simulink model "corr_hw_test"  (R2012b)
settings: Solver=ode45  StartTime=0.0  StopTime=200000  RelTol=1e-3
undefined symbols (not defined in the file or in its folder): gcbh, sfp, xlBlockLoadCallback
libraries: xbsIndex_r4 x1902, casper_library_misc x15, xps_library x6, ox_lib x1
(part 6 of 16)

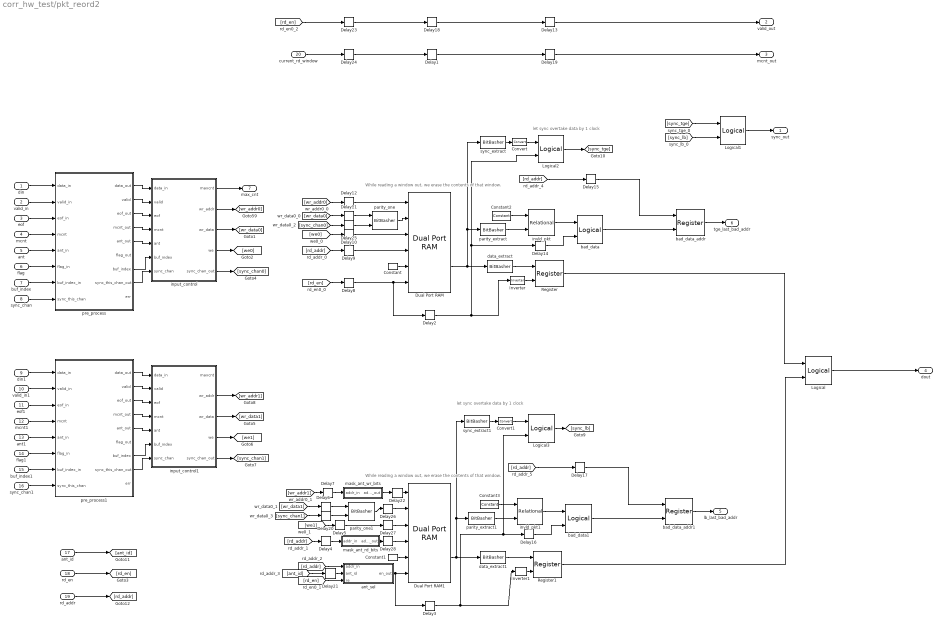
== system corr_hw_test/pkt_reord2 ==
  note: let sync overtake data by 1 clock
  note: While reading a window out,
      | we erase the contents of that window.
  note: While reading a window out,
      | we erase the contents of that window.
  note: let sync overtake data by 1 clock
  din : Inport
  valid_in : Inport  Port=2
  eof : Inport  Port=3
  mcnt : Inport  Port=4
  ant : Inport  Port=5
  flag : Inport  Port=6
  buf_index : Inport  Port=7
  sync_chan : Inport  Port=8
  din1 : Inport  Port=9
  valid_in1 : Inport  Port=10
  eof1 : Inport  Port=11
  mcnt1 : Inport  Port=12
  ant1 : Inport  Port=13
  flag1 : Inport  Port=14
  buf_index1 : Inport  Port=15
  sync_chan1 : Inport  Port=16
  ant_id : Inport  Port=17
  rd_en : Inport  Port=18
  rd_addr : Inport  Port=19
  current_rd_window : Inport  Port=20
  Constant : xbsIndex_r4/Constant  const=0  gui_display_data_type=Fixed-point  arith_type=Unsigned  n_bits=9*(2^x_parallel_bits)  bin_pt=0  preci_type=Single  exp_width=8  frac_width=24  explicit_period=on  period=1  equ=P=C  opselect=C  inp2=PCIN>>17  opr=+  inp1=P  carry=CIN  dbl_ovrd=off  block_type=constant
  Constant1 : xbsIndex_r4/Constant  const=0  gui_display_data_type=Fixed-point  arith_type=Unsigned  n_bits=9*(2^x_parallel_bits)  bin_pt=0  preci_type=Single  exp_width=8  frac_width=24  explicit_period=on  period=1  equ=P=C  opselect=C  inp2=PCIN>>17  opr=+  inp1=P  carry=CIN  dbl_ovrd=off  block_type=constant
  Constant2 : xbsIndex_r4/Constant  const=3  gui_display_data_type=Fixed-point  arith_type=Unsigned  n_bits=2  bin_pt=0  preci_type=Single  exp_width=8  frac_width=24  explicit_period=on  period=1  equ=P=C  opselect=C  inp2=PCIN>>17  opr=+  inp1=P  carry=CIN  dbl_ovrd=off  block_type=constant
  Constant3 : xbsIndex_r4/Constant  const=1  gui_display_data_type=Fixed-point  arith_type=Unsigned  n_bits=1  bin_pt=0  preci_type=Single  exp_width=8  frac_width=24  explicit_period=on  period=1  equ=P=C  opselect=C  inp2=PCIN>>17  opr=+  inp1=P  carry=CIN  dbl_ovrd=off  block_type=constant
  Convert : xbsIndex_r4/Convert  gui_display_data_type=Boolean  arith_type=Boolean  n_bits=3  bin_pt=0  float_type=Single  exp_bits=8  fraction_bits=24  quantization=Truncate  overflow=Wrap  en=off  latency=0  dbl_ovrd=off  pipeline=off  block_type=convert
      settings: block_version=11.4
  Convert1 : xbsIndex_r4/Convert  gui_display_data_type=Boolean  arith_type=Boolean  n_bits=3  bin_pt=0  float_type=Single  exp_bits=8  fraction_bits=24  quantization=Truncate  overflow=Wrap  en=off  latency=0  dbl_ovrd=off  pipeline=off  block_type=convert
      settings: block_version=11.4
  Delay{1..3,18} (4 alike) : xbsIndex_r4/Delay  rst=off  infoeditControl=Selection of Reset will increase slice count due to use of real FFs and instead of SRLs  en=off  latency=3  dbl_ovrd=off  reg_retiming=on  block_type=delay
      settings: xl_area=[0, 0, 0, 0, 0, 0, 0]
  Delay{4..13,19..20,23..25} (15 alike) : xbsIndex_r4/Delay  rst=off  infoeditControl=Selection of Reset will increase slice count due to use of real FFs and instead of SRLs  en=off  latency=1  dbl_ovrd=off  reg_retiming=on  block_type=delay
      settings: xl_area=[0, 0, 0, 0, 0, 0, 0]
  Delay{14,16,21..22,26..28} (7 alike) : xbsIndex_r4/Delay  rst=off  infoeditControl=Selection of Reset will increase slice count due to use of real FFs and instead of SRLs  en=off  latency=1  dbl_ovrd=off  reg_retiming=off  block_type=delay
      settings: xl_area=[0, 0, 0, 0, 0, 0, 0]
  Delay15 : xbsIndex_r4/Delay  rst=off  infoeditControl=Selection of Reset will increase slice count due to use of real FFs and instead of SRLs  en=off  latency=5  dbl_ovrd=off  reg_retiming=on  block_type=delay
      settings: xl_area=[0, 0, 0, 0, 0, 0, 0]
  Delay17 : xbsIndex_r4/Delay  rst=off  infoeditControl=Selection of Reset will increase slice count due to use of real FFs and instead of SRLs  en=off  latency=5  dbl_ovrd=off  reg_retiming=on  block_type=delay
      settings: xl_area=[0, 0, 0, 0, 0, 0, 0]
  Dual Port RAM : xbsIndex_r4/Dual Port RAM  depth=2^x_int_bits * 2^ant_bits * 2^window_bits * 2^(x_parallel_bits - 3)  initVector=1  distributed_mem=Block RAM  init_a=0  init_b=0  rst_a=off  rst_b=off  en_a=off  en_b=off  latency=3  write_mode_A=Read Before Write  write_mode_B=Read Before Write  dbl_ovrd=off  optimize=Area  block_type=dpram
      settings: xl_area=[0, 0, 0, 0, 0, 0, 0]  block_version=10.1.3
  Dual Port RAM1 : xbsIndex_r4/Dual Port RAM  depth=2^x_int_bits * 2^window_bits * 2^(x_parallel_bits - 3)  initVector=1  distributed_mem=Block RAM  init_a=0  init_b=0  rst_a=off  rst_b=off  en_a=off  en_b=off  latency=3  write_mode_A=Read Before Write  write_mode_B=Read Before Write  dbl_ovrd=off  optimize=Area  block_type=dpram
      settings: xl_area=[0, 0, 0, 0, 0, 0, 0]  block_version=10.1.3
  Inverter : xbsIndex_r4/Inverter  en=off  latency=0  dbl_ovrd=off  block_type=inv
  Inverter1 : xbsIndex_r4/Inverter  en=off  latency=0  dbl_ovrd=off  block_type=inv
  Logical : xbsIndex_r4/Logical  logical_function=OR  inputs=2  en=off  latency=0  precision=Full  arith_type=Unsigned  n_bits=16  bin_pt=0  align_bp=on  dbl_ovrd=off  block_type=logical
  Logical1 : xbsIndex_r4/Logical  logical_function=OR  inputs=2  en=off  latency=0  precision=Full  arith_type=Unsigned  n_bits=16  bin_pt=0  align_bp=on  dbl_ovrd=off  block_type=logical
  Logical2 : xbsIndex_r4/Logical  logical_function=AND  inputs=2  en=off  latency=0  precision=Full  arith_type=Unsigned  n_bits=16  bin_pt=0  align_bp=on  dbl_ovrd=off  block_type=logical
  Logical3 : xbsIndex_r4/Logical  logical_function=AND  inputs=2  en=off  latency=0  precision=Full  arith_type=Unsigned  n_bits=16  bin_pt=0  align_bp=on  dbl_ovrd=off  block_type=logical
  Register : xbsIndex_r4/Register  init=0  rst=on  en=off  dbl_ovrd=off  block_type=register
  Register1 : xbsIndex_r4/Register  init=0  rst=on  en=off  dbl_ovrd=off  block_type=register
  ant_sel : Subsystem
  bad_data : xbsIndex_r4/Logical  logical_function=AND  inputs=2  en=off  latency=0  precision=Full  arith_type=Unsigned  n_bits=16  bin_pt=0  align_bp=on  dbl_ovrd=off  block_type=logical
  bad_data1 : xbsIndex_r4/Logical  logical_function=AND  inputs=2  en=off  latency=0  precision=Full  arith_type=Unsigned  n_bits=16  bin_pt=0  align_bp=on  dbl_ovrd=off  block_type=logical
  bad_data_addr : xbsIndex_r4/Register  init=0  rst=off  en=on  dbl_ovrd=off  block_type=register
  bad_data_addr1 : xbsIndex_r4/Register  init=0  rst=off  en=on  dbl_ovrd=off  block_type=register
  data_extract : xbsIndex_r4/BitBasher  bitexpr=|  display_expr=off  sr_1=1  arith_type1=Unsigned  bin_pt1=0  sr_2=2  arith_type2=Unsigned  bin_pt2=0  sr_3=3  arith_type3=Unsigned  bin_pt3=0  sr_4=4  arith_type4=Unsigned  bin_pt4=0  dbl_ovrd=off  block_type=bitbasher
      | <!DOCTYPE HTML PUBLIC "-//W3C//DTD HTML 4.0//EN" "http://www.w3.org/TR/REC-html40/strict.dtd">
      | <html><head><meta name="qrichtext" content="1" /><style type="text/css">
      | p, li { white-space: pre-wrap; }
      | </style></head><body style=" font-family:'Ubuntu'; font-size:11pt; font-weight:400; font-style:normal;">
      | <p style=" margin-top:12px; margin-bottom:12px; margin-left:0px; margin-right:0px; -qt-block-indent:0; text-indent:0px;"><span style=" font-family:'MS Shell Dlg'; font-size:8pt;">out={in[135:72], in[63:0]}</span></p></body></html>
  data_extract1 : xbsIndex_r4/BitBasher  bitexpr=|  display_expr=off  sr_1=1  arith_type1=Unsigned  bin_pt1=0  sr_2=2  arith_type2=Unsigned  bin_pt2=0  sr_3=3  arith_type3=Unsigned  bin_pt3=0  sr_4=4  arith_type4=Unsigned  bin_pt4=0  dbl_ovrd=off  block_type=bitbasher
      | <!DOCTYPE HTML PUBLIC "-//W3C//DTD HTML 4.0//EN" "http://www.w3.org/TR/REC-html40/strict.dtd">
      | <html><head><meta name="qrichtext" content="1" /><style type="text/css">
      | p, li { white-space: pre-wrap; }
      | </style></head><body style=" font-family:'Ubuntu'; font-size:11pt; font-weight:400; font-style:normal;">
      | <p style=" margin-top:12px; margin-bottom:12px; margin-left:0px; margin-right:0px; -qt-block-indent:0; text-indent:0px;"><span style=" font-family:'MS Shell Dlg'; font-size:8pt;">out={in[135:72], in[63:0]}</span></p></body></html>
  input_control : Subsystem
  input_control1 : Subsystem
  invld_pkt : xbsIndex_r4/Relational  mode=a!=b  en=off  latency=1  dbl_ovrd=off  block_type=relational
  invld_pkt1 : xbsIndex_r4/Relational  mode=a!=b  en=off  latency=1  dbl_ovrd=off  block_type=relational
  mask_ant_rd_bits : Subsystem
  mask_ant_wr_bits : Subsystem
  parity_extract : xbsIndex_r4/BitBasher  bitexpr=|  display_expr=off  sr_1=1  arith_type1=Unsigned  bin_pt1=0  sr_2=2  arith_type2=Unsigned  bin_pt2=0  sr_3=3  arith_type3=Unsigned  bin_pt3=0  sr_4=4  arith_type4=Unsigned  bin_pt4=0  dbl_ovrd=off  block_type=bitbasher
      | <!DOCTYPE HTML PUBLIC "-//W3C//DTD HTML 4.0//EN" "http://www.w3.org/TR/REC-html40/strict.dtd">
      | <html><head><meta name="qrichtext" content="1" /><style type="text/css">
      | p, li { white-space: pre-wrap; }
      | </style></head><body style=" font-family:'Ubuntu'; font-size:11pt; font-weight:400; font-style:normal;">
      | <p style=" margin-top:12px; margin-bottom:12px; margin-left:0px; margin-right:0px; -qt-block-indent:0; text-indent:0px;"><span style=" font-family:'MS Shell Dlg'; font-size:8pt;">out={in[143], in[71]}</span></p></body></html>
  parity_extract1 : xbsIndex_r4/BitBasher  bitexpr=|  display_expr=off  sr_1=1  arith_type1=Unsigned  bin_pt1=0  sr_2=2  arith_type2=Unsigned  bin_pt2=0  sr_3=3  arith_type3=Unsigned  bin_pt3=0  sr_4=4  arith_type4=Unsigned  bin_pt4=0  dbl_ovrd=off  block_type=bitbasher
      | <!DOCTYPE HTML PUBLIC "-//W3C//DTD HTML 4.0//EN" "http://www.w3.org/TR/REC-html40/strict.dtd">
      | <html><head><meta name="qrichtext" content="1" /><style type="text/css">
      | p, li { white-space: pre-wrap; }
      | </style></head><body style=" font-family:'Ubuntu'; font-size:11pt; font-weight:400; font-style:normal;">
      | <p style=" margin-top:12px; margin-bottom:12px; margin-left:0px; margin-right:0px; -qt-block-indent:0; text-indent:0px;"><span style=" font-family:'MS Shell Dlg'; font-size:8pt;">out={in[143], in[71]}</span></p></body></html>
  parity_one : xbsIndex_r4/BitBasher  bitexpr=|  display_expr=off  sr_1=1  arith_type1=Unsigned  bin_pt1=0  sr_2=2  arith_type2=Unsigned  bin_pt2=0  sr_3=3  arith_type3=Unsigned  bin_pt3=0  sr_4=4  arith_type4=Unsigned  bin_pt4=0  dbl_ovrd=off  block_type=bitbasher
      | <!DOCTYPE HTML PUBLIC "-//W3C//DTD HTML 4.0//EN" "http://www.w3.org/TR/REC-html40/strict.dtd">
      | <html><head><meta name="qrichtext" content="1" /><style type="text/css">
      | p, li { white-space: pre-wrap; }
      | </style></head><body style=" font-family:'Ubuntu'; font-size:11pt; font-weight:400; font-style:normal;">
      | <p style=" margin-top:12px; margin-bottom:12px; margin-left:0px; margin-right:0px; -qt-block-indent:0; text-indent:0px;"><span style=" font-family:'MS Shell Dlg'; font-size:8pt;">out={1'b1, sync_chan, 6'b0, data[63:0]}</span></p></body></html>
  parity_one1 : xbsIndex_r4/BitBasher  bitexpr=|  display_expr=off  sr_1=1  arith_type1=Unsigned  bin_pt1=0  sr_2=2  arith_type2=Unsigned  bin_pt2=0  sr_3=3  arith_type3=Unsigned  bin_pt3=0  sr_4=4  arith_type4=Unsigned  bin_pt4=0  dbl_ovrd=off  block_type=bitbasher
      | <!DOCTYPE HTML PUBLIC "-//W3C//DTD HTML 4.0//EN" "http://www.w3.org/TR/REC-html40/strict.dtd">
      | <html><head><meta name="qrichtext" content="1" /><style type="text/css">
      | p, li { white-space: pre-wrap; }
      | </style></head><body style=" font-family:'Ubuntu'; font-size:11pt; font-weight:400; font-style:normal;">
      | <p style=" margin-top:12px; margin-bottom:12px; margin-left:0px; margin-right:0px; -qt-block-indent:0; text-indent:0px;"><span style=" font-family:'MS Shell Dlg'; font-size:8pt;">out={1'b1, sync_chan, 6'b0, data[63:0]}</span></p></body></html>
  pre_process : Subsystem
  pre_process1 : Subsystem
  sync_extract : xbsIndex_r4/BitBasher  bitexpr=|  display_expr=off  sr_1=1  arith_type1=Unsigned  bin_pt1=0  sr_2=2  arith_type2=Unsigned  bin_pt2=0  sr_3=3  arith_type3=Unsigned  bin_pt3=0  sr_4=4  arith_type4=Unsigned  bin_pt4=0  dbl_ovrd=off  block_type=bitbasher
      | <!DOCTYPE HTML PUBLIC "-//W3C//DTD HTML 4.0//EN" "http://www.w3.org/TR/REC-html40/strict.dtd">
      | <html><head><meta name="qrichtext" content="1" /><style type="text/css">
      | p, li { white-space: pre-wrap; }
      | </style></head><body style=" font-family:'Ubuntu'; font-size:11pt; font-weight:400; font-style:normal;">
      | <p style=" margin-top:12px; margin-bottom:12px; margin-left:0px; margin-right:0px; -qt-block-indent:0; text-indent:0px;"><span style=" font-family:'MS Shell Dlg'; font-size:8pt;">out={in[64]}</span></p></body></html>
  sync_extract1 : xbsIndex_r4/BitBasher  bitexpr=|  display_expr=off  sr_1=1  arith_type1=Unsigned  bin_pt1=0  sr_2=2  arith_type2=Unsigned  bin_pt2=0  sr_3=3  arith_type3=Unsigned  bin_pt3=0  sr_4=4  arith_type4=Unsigned  bin_pt4=0  dbl_ovrd=off  block_type=bitbasher
      | <!DOCTYPE HTML PUBLIC "-//W3C//DTD HTML 4.0//EN" "http://www.w3.org/TR/REC-html40/strict.dtd">
      | <html><head><meta name="qrichtext" content="1" /><style type="text/css">
      | p, li { white-space: pre-wrap; }
      | </style></head><body style=" font-family:'Ubuntu'; font-size:11pt; font-weight:400; font-style:normal;">
      | <p style=" margin-top:12px; margin-bottom:12px; margin-left:0px; margin-right:0px; -qt-block-indent:0; text-indent:0px;"><span style=" font-family:'MS Shell Dlg'; font-size:8pt;">out={in[64]}</span></p></body></html>
  sync_out : Outport
  valid_out : Outport  Port=2
  mcnt_out : Outport  Port=3
  dout : Outport  Port=4
  lb_last_bad_addr : Outport  Port=5
  tge_last_bad_addr : Outport  Port=6
  max_cnt : Outport  Port=7
  wires:
  Delay1/1 -> Delay19/1
  input_control/3(wr_data) -> [wr_data0]
  Delay13/1 -> valid_out/1
  input_control/2(wr_addr) -> [wr_addr0]
  input_control/4(we) -> [we0]
  valid_in/1 -> pre_process/2(valid_in)
  mcnt/1 -> pre_process/4(mcnt)
  din/1 -> pre_process/1(data_in)
  eof/1 -> pre_process/3(eof_in)
  ant/1 -> pre_process/5(ant_in)
  flag/1 -> pre_process/6(flag_in)
  pre_process/1(data_out) -> input_control/1(data_in)
  pre_process/2(valid) -> input_control/2(valid)
  pre_process/3(eof_out) -> input_control/3(eof)
  pre_process/4(mcnt_out) -> input_control/4(mcnt)
  pre_process/5(ant_out) -> input_control/5(ant)
  pre_process/7(buf_index) -> input_control/6(buf_index)
  buf_index/1 -> pre_process/7(buf_index_in)
  Constant/1 -> Dual Port RAM/5
  [wr_addr0] -> Delay12/1
  [we0] -> Delay10/1
  [wr_data0] -> Delay11/1
  [rd_addr] -> Delay9/1
  [rd_en] -> Delay8/1
  Dual Port RAM/2 -> data_extract/1, sync_extract/1, parity_extract/1
  Delay2/1 -> Logical2/2, Delay14/1, Inverter/1
  Inverter/1 -> Register/2
  Constant1/1 -> Dual Port RAM1/5
  [wr_addr1] -> Delay7/1
  [we1] -> Delay5/1
  [rd_addr] -> Delay4/1
  Dual Port RAM1/2 -> parity_extract1/1, sync_extract1/1, data_extract1/1
  Delay3/1 -> Delay16/1, Logical3/2, Inverter1/1
  Inverter1/1 -> Register1/2
  mask_ant_wr_bits/1(addr_out) -> Delay22/1
  mask_ant_rd_bits/1(addr_out) -> Delay28/1
  [rd_en] -> ant_sel/3(re)
  [rd_addr] -> ant_sel/1(addr_in)
  [ant_id] -> Delay21/1
  ant_id/1 -> [ant_id]
  ant_sel/1(en_out) -> Delay3/1, Dual Port RAM1/6
  Delay4/1 -> mask_ant_rd_bits/1(addr_in)
  Delay5/1 -> Delay27/1
  Delay7/1 -> mask_ant_wr_bits/1(addr_in)
  Delay8/1 -> Delay2/1, Dual Port RAM/6
  Delay9/1 -> Dual Port RAM/4
  Delay10/1 -> Dual Port RAM/3
  Delay12/1 -> Dual Port RAM/1
  Register/1 -> Logical/1
  Register1/1 -> Logical/2
  Logical/1 -> dout/1
  [rd_en] -> Delay23/1
  rd_en/1 -> [rd_en]
  rd_addr/1 -> [rd_addr]
  Delay11/1 -> parity_one/1
  parity_one/1 -> Dual Port RAM/2
  data_extract/1 -> Register/1
  data_extract1/1 -> Register1/1
  parity_extract/1 -> invld_pkt/2
  Constant2/1 -> invld_pkt/1
  Delay14/1 -> bad_data/2
  invld_pkt/1 -> bad_data/1
  bad_data/1 -> bad_data_addr/2
  [rd_addr] -> Delay15/1
  Delay15/1 -> bad_data_addr/1
  parity_extract1/1 -> invld_pkt1/2
  Constant3/1 -> invld_pkt1/1
  Delay16/1 -> bad_data1/2
  invld_pkt1/1 -> bad_data1/1
  bad_data1/1 -> bad_data_addr1/2
  [rd_addr] -> Delay17/1
  Delay17/1 -> bad_data_addr1/1
  bad_data_addr1/1 -> lb_last_bad_addr/1
  bad_data_addr/1 -> tge_last_bad_addr/1
  current_rd_window/1 -> Delay24/1
  input_control/1(maxcnt) -> max_cnt/1
  Delay18/1 -> Delay13/1
  Delay19/1 -> mcnt_out/1
  Delay23/1 -> Delay18/1
  Delay24/1 -> Delay1/1
  sync_chan/1 -> pre_process/8(sync_this_chan)
  pre_process/8(sync_this_chan_out) -> input_control/7(sync_chan)
  input_control/5(sync_chan_out) -> [sync_chan0]
  [sync_chan0] -> Delay25/1
  Delay25/1 -> parity_one/2
  input_control1/3(wr_data) -> [wr_data1]
  input_control1/2(wr_addr) -> [wr_addr1]
  input_control1/4(we) -> [we1]
  valid_in1/1 -> pre_process1/2(valid_in)
  mcnt1/1 -> pre_process1/4(mcnt)
  din1/1 -> pre_process1/1(data_in)
  eof1/1 -> pre_process1/3(eof_in)
  ant1/1 -> pre_process1/5(ant_in)
  flag1/1 -> pre_process1/6(flag_in)
  pre_process1/1(data_out) -> input_control1/1(data_in)
  pre_process1/2(valid) -> input_control1/2(valid)
  pre_process1/3(eof_out) -> input_control1/3(eof)
  pre_process1/4(mcnt_out) -> input_control1/4(mcnt)
  pre_process1/5(ant_out) -> input_control1/5(ant)
  pre_process1/7(buf_index) -> input_control1/6(buf_index)
  buf_index1/1 -> pre_process1/7(buf_index_in)
  sync_chan1/1 -> pre_process1/8(sync_this_chan)
  pre_process1/8(sync_this_chan_out) -> input_control1/7(sync_chan)
  input_control1/5(sync_chan_out) -> [sync_chan1]
  [wr_data1] -> Delay6/1
  Delay6/1 -> parity_one1/1
  [sync_chan1] -> Delay20/1
  Delay20/1 -> parity_one1/2
  parity_one1/1 -> Delay26/1
  [sync_tge] -> Logical1/1
  [sync_lb] -> Logical1/2
  Logical1/1 -> sync_out/1
  sync_extract/1 -> Convert/1
  Logical2/1 -> [sync_tge]
  sync_extract1/1 -> Convert1/1
  Logical3/1 -> [sync_lb]
  Convert/1 -> Logical2/1
  Convert1/1 -> Logical3/1
  Delay21/1 -> ant_sel/2(ant_id)
  Delay22/1 -> Dual Port RAM1/1
  Delay26/1 -> Dual Port RAM1/2
  Delay27/1 -> Dual Port RAM1/3
  Delay28/1 -> Dual Port RAM1/4

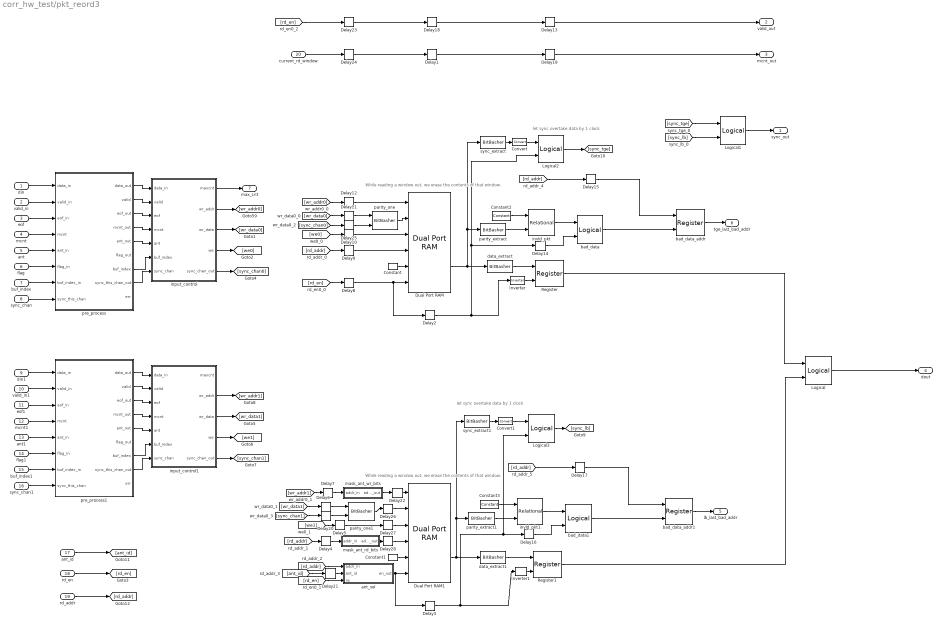
== system corr_hw_test/pkt_reord3 ==
  note: let sync overtake data by 1 clock
  note: While reading a window out,
      | we erase the contents of that window.
  note: While reading a window out,
      | we erase the contents of that window.
  note: let sync overtake data by 1 clock
  din : Inport
  valid_in : Inport  Port=2
  eof : Inport  Port=3
  mcnt : Inport  Port=4
  ant : Inport  Port=5
  flag : Inport  Port=6
  buf_index : Inport  Port=7
  sync_chan : Inport  Port=8
  din1 : Inport  Port=9
  valid_in1 : Inport  Port=10
  eof1 : Inport  Port=11
  mcnt1 : Inport  Port=12
  ant1 : Inport  Port=13
  flag1 : Inport  Port=14
  buf_index1 : Inport  Port=15
  sync_chan1 : Inport  Port=16
  ant_id : Inport  Port=17
  rd_en : Inport  Port=18
  rd_addr : Inport  Port=19
  current_rd_window : Inport  Port=20
  Constant : xbsIndex_r4/Constant  const=0  gui_display_data_type=Fixed-point  arith_type=Unsigned  n_bits=9*(2^x_parallel_bits)  bin_pt=0  preci_type=Single  exp_width=8  frac_width=24  explicit_period=on  period=1  equ=P=C  opselect=C  inp2=PCIN>>17  opr=+  inp1=P  carry=CIN  dbl_ovrd=off  block_type=constant
  Constant1 : xbsIndex_r4/Constant  const=0  gui_display_data_type=Fixed-point  arith_type=Unsigned  n_bits=9*(2^x_parallel_bits)  bin_pt=0  preci_type=Single  exp_width=8  frac_width=24  explicit_period=on  period=1  equ=P=C  opselect=C  inp2=PCIN>>17  opr=+  inp1=P  carry=CIN  dbl_ovrd=off  block_type=constant
  Constant2 : xbsIndex_r4/Constant  const=3  gui_display_data_type=Fixed-point  arith_type=Unsigned  n_bits=2  bin_pt=0  preci_type=Single  exp_width=8  frac_width=24  explicit_period=on  period=1  equ=P=C  opselect=C  inp2=PCIN>>17  opr=+  inp1=P  carry=CIN  dbl_ovrd=off  block_type=constant
  Constant3 : xbsIndex_r4/Constant  const=1  gui_display_data_type=Fixed-point  arith_type=Unsigned  n_bits=1  bin_pt=0  preci_type=Single  exp_width=8  frac_width=24  explicit_period=on  period=1  equ=P=C  opselect=C  inp2=PCIN>>17  opr=+  inp1=P  carry=CIN  dbl_ovrd=off  block_type=constant
  Convert : xbsIndex_r4/Convert  gui_display_data_type=Boolean  arith_type=Boolean  n_bits=3  bin_pt=0  float_type=Single  exp_bits=8  fraction_bits=24  quantization=Truncate  overflow=Wrap  en=off  latency=0  dbl_ovrd=off  pipeline=off  block_type=convert
      settings: block_version=11.4
  Convert1 : xbsIndex_r4/Convert  gui_display_data_type=Boolean  arith_type=Boolean  n_bits=3  bin_pt=0  float_type=Single  exp_bits=8  fraction_bits=24  quantization=Truncate  overflow=Wrap  en=off  latency=0  dbl_ovrd=off  pipeline=off  block_type=convert
      settings: block_version=11.4
  Delay{1..3,18} (4 alike) : xbsIndex_r4/Delay  rst=off  infoeditControl=Selection of Reset will increase slice count due to use of real FFs and instead of SRLs  en=off  latency=3  dbl_ovrd=off  reg_retiming=on  block_type=delay
      settings: xl_area=[0, 0, 0, 0, 0, 0, 0]
  Delay{4..13,19..20,23..25} (15 alike) : xbsIndex_r4/Delay  rst=off  infoeditControl=Selection of Reset will increase slice count due to use of real FFs and instead of SRLs  en=off  latency=1  dbl_ovrd=off  reg_retiming=on  block_type=delay
      settings: xl_area=[0, 0, 0, 0, 0, 0, 0]
  Delay{14,16,21..22,26..28} (7 alike) : xbsIndex_r4/Delay  rst=off  infoeditControl=Selection of Reset will increase slice count due to use of real FFs and instead of SRLs  en=off  latency=1  dbl_ovrd=off  reg_retiming=off  block_type=delay
      settings: xl_area=[0, 0, 0, 0, 0, 0, 0]
  Delay15 : xbsIndex_r4/Delay  rst=off  infoeditControl=Selection of Reset will increase slice count due to use of real FFs and instead of SRLs  en=off  latency=5  dbl_ovrd=off  reg_retiming=on  block_type=delay
      settings: xl_area=[0, 0, 0, 0, 0, 0, 0]
  Delay17 : xbsIndex_r4/Delay  rst=off  infoeditControl=Selection of Reset will increase slice count due to use of real FFs and instead of SRLs  en=off  latency=5  dbl_ovrd=off  reg_retiming=on  block_type=delay
      settings: xl_area=[0, 0, 0, 0, 0, 0, 0]
  Dual Port RAM : xbsIndex_r4/Dual Port RAM  depth=2^x_int_bits * 2^ant_bits * 2^window_bits * 2^(x_parallel_bits - 3)  initVector=1  distributed_mem=Block RAM  init_a=0  init_b=0  rst_a=off  rst_b=off  en_a=off  en_b=off  latency=3  write_mode_A=Read Before Write  write_mode_B=Read Before Write  dbl_ovrd=off  optimize=Area  block_type=dpram
      settings: xl_area=[0, 0, 0, 0, 0, 0, 0]  block_version=10.1.3
  Dual Port RAM1 : xbsIndex_r4/Dual Port RAM  depth=2^x_int_bits * 2^window_bits * 2^(x_parallel_bits - 3)  initVector=1  distributed_mem=Block RAM  init_a=0  init_b=0  rst_a=off  rst_b=off  en_a=off  en_b=off  latency=3  write_mode_A=Read Before Write  write_mode_B=Read Before Write  dbl_ovrd=off  optimize=Area  block_type=dpram
      settings: xl_area=[0, 0, 0, 0, 0, 0, 0]  block_version=10.1.3
  Inverter : xbsIndex_r4/Inverter  en=off  latency=0  dbl_ovrd=off  block_type=inv
  Inverter1 : xbsIndex_r4/Inverter  en=off  latency=0  dbl_ovrd=off  block_type=inv
  Logical : xbsIndex_r4/Logical  logical_function=OR  inputs=2  en=off  latency=0  precision=Full  arith_type=Unsigned  n_bits=16  bin_pt=0  align_bp=on  dbl_ovrd=off  block_type=logical
  Logical1 : xbsIndex_r4/Logical  logical_function=OR  inputs=2  en=off  latency=0  precision=Full  arith_type=Unsigned  n_bits=16  bin_pt=0  align_bp=on  dbl_ovrd=off  block_type=logical
  Logical2 : xbsIndex_r4/Logical  logical_function=AND  inputs=2  en=off  latency=0  precision=Full  arith_type=Unsigned  n_bits=16  bin_pt=0  align_bp=on  dbl_ovrd=off  block_type=logical
  Logical3 : xbsIndex_r4/Logical  logical_function=AND  inputs=2  en=off  latency=0  precision=Full  arith_type=Unsigned  n_bits=16  bin_pt=0  align_bp=on  dbl_ovrd=off  block_type=logical
  Register : xbsIndex_r4/Register  init=0  rst=on  en=off  dbl_ovrd=off  block_type=register
  Register1 : xbsIndex_r4/Register  init=0  rst=on  en=off  dbl_ovrd=off  block_type=register
  ant_sel : Subsystem
  bad_data : xbsIndex_r4/Logical  logical_function=AND  inputs=2  en=off  latency=0  precision=Full  arith_type=Unsigned  n_bits=16  bin_pt=0  align_bp=on  dbl_ovrd=off  block_type=logical
  bad_data1 : xbsIndex_r4/Logical  logical_function=AND  inputs=2  en=off  latency=0  precision=Full  arith_type=Unsigned  n_bits=16  bin_pt=0  align_bp=on  dbl_ovrd=off  block_type=logical
  bad_data_addr : xbsIndex_r4/Register  init=0  rst=off  en=on  dbl_ovrd=off  block_type=register
  bad_data_addr1 : xbsIndex_r4/Register  init=0  rst=off  en=on  dbl_ovrd=off  block_type=register
  data_extract : xbsIndex_r4/BitBasher  bitexpr=|  display_expr=off  sr_1=1  arith_type1=Unsigned  bin_pt1=0  sr_2=2  arith_type2=Unsigned  bin_pt2=0  sr_3=3  arith_type3=Unsigned  bin_pt3=0  sr_4=4  arith_type4=Unsigned  bin_pt4=0  dbl_ovrd=off  block_type=bitbasher
      | <!DOCTYPE HTML PUBLIC "-//W3C//DTD HTML 4.0//EN" "http://www.w3.org/TR/REC-html40/strict.dtd">
      | <html><head><meta name="qrichtext" content="1" /><style type="text/css">
      | p, li { white-space: pre-wrap; }
      | </style></head><body style=" font-family:'Ubuntu'; font-size:11pt; font-weight:400; font-style:normal;">
      | <p style=" margin-top:12px; margin-bottom:12px; margin-left:0px; margin-right:0px; -qt-block-indent:0; text-indent:0px;"><span style=" font-family:'MS Shell Dlg'; font-size:8pt;">out={in[135:72], in[63:0]}</span></p></body></html>
  data_extract1 : xbsIndex_r4/BitBasher  bitexpr=|  display_expr=off  sr_1=1  arith_type1=Unsigned  bin_pt1=0  sr_2=2  arith_type2=Unsigned  bin_pt2=0  sr_3=3  arith_type3=Unsigned  bin_pt3=0  sr_4=4  arith_type4=Unsigned  bin_pt4=0  dbl_ovrd=off  block_type=bitbasher
      | <!DOCTYPE HTML PUBLIC "-//W3C//DTD HTML 4.0//EN" "http://www.w3.org/TR/REC-html40/strict.dtd">
      | <html><head><meta name="qrichtext" content="1" /><style type="text/css">
      | p, li { white-space: pre-wrap; }
      | </style></head><body style=" font-family:'Ubuntu'; font-size:11pt; font-weight:400; font-style:normal;">
      | <p style=" margin-top:12px; margin-bottom:12px; margin-left:0px; margin-right:0px; -qt-block-indent:0; text-indent:0px;"><span style=" font-family:'MS Shell Dlg'; font-size:8pt;">out={in[135:72], in[63:0]}</span></p></body></html>
  input_control : Subsystem
  input_control1 : Subsystem
  invld_pkt : xbsIndex_r4/Relational  mode=a!=b  en=off  latency=1  dbl_ovrd=off  block_type=relational
  invld_pkt1 : xbsIndex_r4/Relational  mode=a!=b  en=off  latency=1  dbl_ovrd=off  block_type=relational
  mask_ant_rd_bits : Subsystem
  mask_ant_wr_bits : Subsystem
  parity_extract : xbsIndex_r4/BitBasher  bitexpr=|  display_expr=off  sr_1=1  arith_type1=Unsigned  bin_pt1=0  sr_2=2  arith_type2=Unsigned  bin_pt2=0  sr_3=3  arith_type3=Unsigned  bin_pt3=0  sr_4=4  arith_type4=Unsigned  bin_pt4=0  dbl_ovrd=off  block_type=bitbasher
      | <!DOCTYPE HTML PUBLIC "-//W3C//DTD HTML 4.0//EN" "http://www.w3.org/TR/REC-html40/strict.dtd">
      | <html><head><meta name="qrichtext" content="1" /><style type="text/css">
      | p, li { white-space: pre-wrap; }
      | </style></head><body style=" font-family:'Ubuntu'; font-size:11pt; font-weight:400; font-style:normal;">
      | <p style=" margin-top:12px; margin-bottom:12px; margin-left:0px; margin-right:0px; -qt-block-indent:0; text-indent:0px;"><span style=" font-family:'MS Shell Dlg'; font-size:8pt;">out={in[143], in[71]}</span></p></body></html>
  parity_extract1 : xbsIndex_r4/BitBasher  bitexpr=|  display_expr=off  sr_1=1  arith_type1=Unsigned  bin_pt1=0  sr_2=2  arith_type2=Unsigned  bin_pt2=0  sr_3=3  arith_type3=Unsigned  bin_pt3=0  sr_4=4  arith_type4=Unsigned  bin_pt4=0  dbl_ovrd=off  block_type=bitbasher
      | <!DOCTYPE HTML PUBLIC "-//W3C//DTD HTML 4.0//EN" "http://www.w3.org/TR/REC-html40/strict.dtd">
      | <html><head><meta name="qrichtext" content="1" /><style type="text/css">
      | p, li { white-space: pre-wrap; }
      | </style></head><body style=" font-family:'Ubuntu'; font-size:11pt; font-weight:400; font-style:normal;">
      | <p style=" margin-top:12px; margin-bottom:12px; margin-left:0px; margin-right:0px; -qt-block-indent:0; text-indent:0px;"><span style=" font-family:'MS Shell Dlg'; font-size:8pt;">out={in[143], in[71]}</span></p></body></html>
  parity_one : xbsIndex_r4/BitBasher  bitexpr=|  display_expr=off  sr_1=1  arith_type1=Unsigned  bin_pt1=0  sr_2=2  arith_type2=Unsigned  bin_pt2=0  sr_3=3  arith_type3=Unsigned  bin_pt3=0  sr_4=4  arith_type4=Unsigned  bin_pt4=0  dbl_ovrd=off  block_type=bitbasher
      | <!DOCTYPE HTML PUBLIC "-//W3C//DTD HTML 4.0//EN" "http://www.w3.org/TR/REC-html40/strict.dtd">
      | <html><head><meta name="qrichtext" content="1" /><style type="text/css">
      | p, li { white-space: pre-wrap; }
      | </style></head><body style=" font-family:'Ubuntu'; font-size:11pt; font-weight:400; font-style:normal;">
      | <p style=" margin-top:12px; margin-bottom:12px; margin-left:0px; margin-right:0px; -qt-block-indent:0; text-indent:0px;"><span style=" font-family:'MS Shell Dlg'; font-size:8pt;">out={1'b1, sync_chan, 6'b0, data[63:0]}</span></p></body></html>
  parity_one1 : xbsIndex_r4/BitBasher  bitexpr=|  display_expr=off  sr_1=1  arith_type1=Unsigned  bin_pt1=0  sr_2=2  arith_type2=Unsigned  bin_pt2=0  sr_3=3  arith_type3=Unsigned  bin_pt3=0  sr_4=4  arith_type4=Unsigned  bin_pt4=0  dbl_ovrd=off  block_type=bitbasher
      | <!DOCTYPE HTML PUBLIC "-//W3C//DTD HTML 4.0//EN" "http://www.w3.org/TR/REC-html40/strict.dtd">
      | <html><head><meta name="qrichtext" content="1" /><style type="text/css">
      | p, li { white-space: pre-wrap; }
      | </style></head><body style=" font-family:'Ubuntu'; font-size:11pt; font-weight:400; font-style:normal;">
      | <p style=" margin-top:12px; margin-bottom:12px; margin-left:0px; margin-right:0px; -qt-block-indent:0; text-indent:0px;"><span style=" font-family:'MS Shell Dlg'; font-size:8pt;">out={1'b1, sync_chan, 6'b0, data[63:0]}</span></p></body></html>
  pre_process : Subsystem
  pre_process1 : Subsystem
  sync_extract : xbsIndex_r4/BitBasher  bitexpr=|  display_expr=off  sr_1=1  arith_type1=Unsigned  bin_pt1=0  sr_2=2  arith_type2=Unsigned  bin_pt2=0  sr_3=3  arith_type3=Unsigned  bin_pt3=0  sr_4=4  arith_type4=Unsigned  bin_pt4=0  dbl_ovrd=off  block_type=bitbasher
      | <!DOCTYPE HTML PUBLIC "-//W3C//DTD HTML 4.0//EN" "http://www.w3.org/TR/REC-html40/strict.dtd">
      | <html><head><meta name="qrichtext" content="1" /><style type="text/css">
      | p, li { white-space: pre-wrap; }
      | </style></head><body style=" font-family:'Ubuntu'; font-size:11pt; font-weight:400; font-style:normal;">
      | <p style=" margin-top:12px; margin-bottom:12px; margin-left:0px; margin-right:0px; -qt-block-indent:0; text-indent:0px;"><span style=" font-family:'MS Shell Dlg'; font-size:8pt;">out={in[64]}</span></p></body></html>
  sync_extract1 : xbsIndex_r4/BitBasher  bitexpr=|  display_expr=off  sr_1=1  arith_type1=Unsigned  bin_pt1=0  sr_2=2  arith_type2=Unsigned  bin_pt2=0  sr_3=3  arith_type3=Unsigned  bin_pt3=0  sr_4=4  arith_type4=Unsigned  bin_pt4=0  dbl_ovrd=off  block_type=bitbasher
      | <!DOCTYPE HTML PUBLIC "-//W3C//DTD HTML 4.0//EN" "http://www.w3.org/TR/REC-html40/strict.dtd">
      | <html><head><meta name="qrichtext" content="1" /><style type="text/css">
      | p, li { white-space: pre-wrap; }
      | </style></head><body style=" font-family:'Ubuntu'; font-size:11pt; font-weight:400; font-style:normal;">
      | <p style=" margin-top:12px; margin-bottom:12px; margin-left:0px; margin-right:0px; -qt-block-indent:0; text-indent:0px;"><span style=" font-family:'MS Shell Dlg'; font-size:8pt;">out={in[64]}</span></p></body></html>
  sync_out : Outport
  valid_out : Outport  Port=2
  mcnt_out : Outport  Port=3
  dout : Outport  Port=4
  lb_last_bad_addr : Outport  Port=5
  tge_last_bad_addr : Outport  Port=6
  max_cnt : Outport  Port=7
  wires:
  Delay28/1 -> Dual Port RAM1/4
  Delay27/1 -> Dual Port RAM1/3
  Delay26/1 -> Dual Port RAM1/2
  Delay22/1 -> Dual Port RAM1/1
  Delay21/1 -> ant_sel/2(ant_id)
  Convert1/1 -> Logical3/1
  Convert/1 -> Logical2/1
  Logical3/1 -> [sync_lb]
  sync_extract1/1 -> Convert1/1
  Logical2/1 -> [sync_tge]
  sync_extract/1 -> Convert/1
  Logical1/1 -> sync_out/1
  [sync_lb] -> Logical1/2
  [sync_tge] -> Logical1/1
  parity_one1/1 -> Delay26/1
  Delay20/1 -> parity_one1/2
  [sync_chan1] -> Delay20/1
  Delay6/1 -> parity_one1/1
  [wr_data1] -> Delay6/1
  input_control1/5(sync_chan_out) -> [sync_chan1]
  pre_process1/8(sync_this_chan_out) -> input_control1/7(sync_chan)
  sync_chan1/1 -> pre_process1/8(sync_this_chan)
  buf_index1/1 -> pre_process1/7(buf_index_in)
  pre_process1/7(buf_index) -> input_control1/6(buf_index)
  pre_process1/5(ant_out) -> input_control1/5(ant)
  pre_process1/4(mcnt_out) -> input_control1/4(mcnt)
  pre_process1/3(eof_out) -> input_control1/3(eof)
  pre_process1/2(valid) -> input_control1/2(valid)
  pre_process1/1(data_out) -> input_control1/1(data_in)
  flag1/1 -> pre_process1/6(flag_in)
  ant1/1 -> pre_process1/5(ant_in)
  eof1/1 -> pre_process1/3(eof_in)
  din1/1 -> pre_process1/1(data_in)
  mcnt1/1 -> pre_process1/4(mcnt)
  valid_in1/1 -> pre_process1/2(valid_in)
  input_control1/4(we) -> [we1]
  input_control1/2(wr_addr) -> [wr_addr1]
  input_control1/3(wr_data) -> [wr_data1]
  Delay25/1 -> parity_one/2
  [sync_chan0] -> Delay25/1
  input_control/5(sync_chan_out) -> [sync_chan0]
  pre_process/8(sync_this_chan_out) -> input_control/7(sync_chan)
  sync_chan/1 -> pre_process/8(sync_this_chan)
  Delay24/1 -> Delay1/1
  Delay23/1 -> Delay18/1
  Delay19/1 -> mcnt_out/1
  Delay18/1 -> Delay13/1
  input_control/1(maxcnt) -> max_cnt/1
  current_rd_window/1 -> Delay24/1
  bad_data_addr/1 -> tge_last_bad_addr/1
  bad_data_addr1/1 -> lb_last_bad_addr/1
  Delay17/1 -> bad_data_addr1/1
  [rd_addr] -> Delay17/1
  bad_data1/1 -> bad_data_addr1/2
  invld_pkt1/1 -> bad_data1/1
  Delay16/1 -> bad_data1/2
  Constant3/1 -> invld_pkt1/1
  parity_extract1/1 -> invld_pkt1/2
  Delay15/1 -> bad_data_addr/1
  [rd_addr] -> Delay15/1
  bad_data/1 -> bad_data_addr/2
  invld_pkt/1 -> bad_data/1
  Delay14/1 -> bad_data/2
  Constant2/1 -> invld_pkt/1
  parity_extract/1 -> invld_pkt/2
  data_extract1/1 -> Register1/1
  data_extract/1 -> Register/1
  parity_one/1 -> Dual Port RAM/2
  Delay11/1 -> parity_one/1
  rd_addr/1 -> [rd_addr]
  rd_en/1 -> [rd_en]
  [rd_en] -> Delay23/1
  Logical/1 -> dout/1
  Register1/1 -> Logical/2
  Register/1 -> Logical/1
  Delay12/1 -> Dual Port RAM/1
  Delay10/1 -> Dual Port RAM/3
  Delay9/1 -> Dual Port RAM/4
  Delay8/1 -> Dual Port RAM/6, Delay2/1
  Delay7/1 -> mask_ant_wr_bits/1(addr_in)
  Delay5/1 -> Delay27/1
  Delay4/1 -> mask_ant_rd_bits/1(addr_in)
  ant_sel/1(en_out) -> Dual Port RAM1/6, Delay3/1
  ant_id/1 -> [ant_id]
  [ant_id] -> Delay21/1
  [rd_addr] -> ant_sel/1(addr_in)
  [rd_en] -> ant_sel/3(re)
  mask_ant_rd_bits/1(addr_out) -> Delay28/1
  mask_ant_wr_bits/1(addr_out) -> Delay22/1
  Inverter1/1 -> Register1/2
  Delay3/1 -> Inverter1/1, Logical3/2, Delay16/1
  Dual Port RAM1/2 -> data_extract1/1, sync_extract1/1, parity_extract1/1
  [rd_addr] -> Delay4/1
  [we1] -> Delay5/1
  [wr_addr1] -> Delay7/1
  Constant1/1 -> Dual Port RAM1/5
  Inverter/1 -> Register/2
  Delay2/1 -> Inverter/1, Delay14/1, Logical2/2
  Dual Port RAM/2 -> parity_extract/1, sync_extract/1, data_extract/1
  [rd_en] -> Delay8/1
  [rd_addr] -> Delay9/1
  [wr_data0] -> Delay11/1
  [we0] -> Delay10/1
  [wr_addr0] -> Delay12/1
  Constant/1 -> Dual Port RAM/5
  buf_index/1 -> pre_process/7(buf_index_in)
  pre_process/7(buf_index) -> input_control/6(buf_index)
  pre_process/5(ant_out) -> input_control/5(ant)
  pre_process/4(mcnt_out) -> input_control/4(mcnt)
  pre_process/3(eof_out) -> input_control/3(eof)
  pre_process/2(valid) -> input_control/2(valid)
  pre_process/1(data_out) -> input_control/1(data_in)
  flag/1 -> pre_process/6(flag_in)
  ant/1 -> pre_process/5(ant_in)
  eof/1 -> pre_process/3(eof_in)
  din/1 -> pre_process/1(data_in)
  mcnt/1 -> pre_process/4(mcnt)
  valid_in/1 -> pre_process/2(valid_in)
  input_control/4(we) -> [we0]
  input_control/2(wr_addr) -> [wr_addr0]
  Delay13/1 -> valid_out/1
  input_control/3(wr_data) -> [wr_data0]
  Delay1/1 -> Delay19/1
